simulink model "main"  (R2025b)
settings: Solver=ode4  StartTime=0.0  StopTime=60  FixedStep=Ts_inner  RelTol=1e-3
undefined symbols (not defined in the file): Ts_gcs
libraries: aerolibutil x4, instrumentseriallib x2, sldrtlib x1
settings Model: DataDictionary=project.sldd  Creator=Nick  LastModifiedBy=Nick
settings SolverCC: AutoInsertRateTranBlk=on

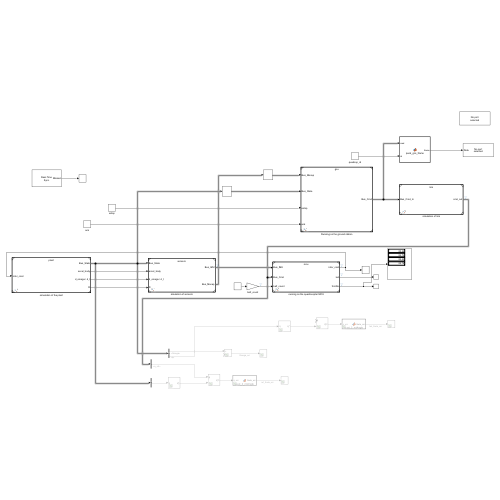
[thumbnail: Simulink's stored preview of the top-level diagram]
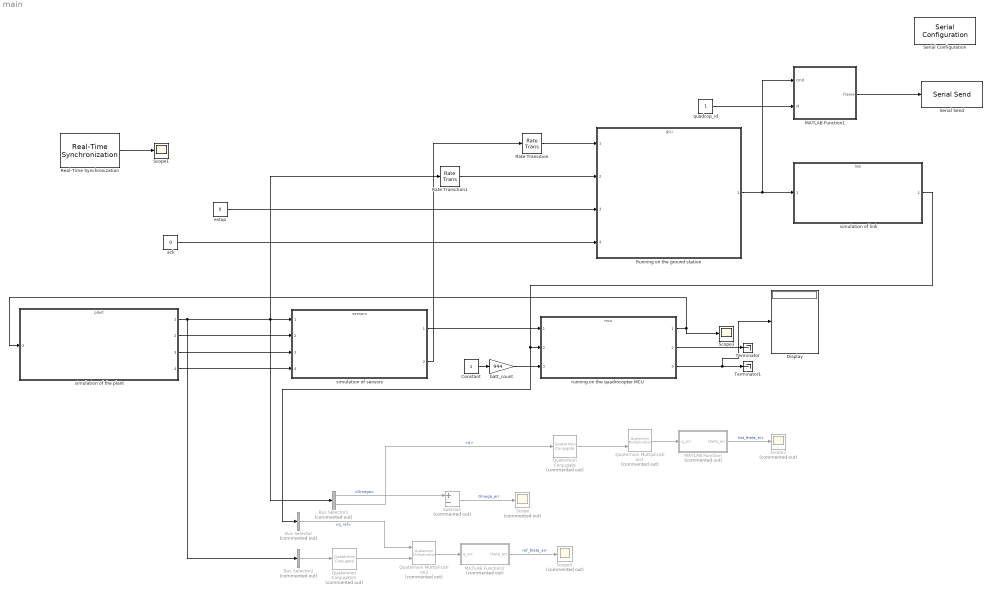
== system main ==
  Bus Selector : BusSelector  Commented=on  OutputSignals=q_ref
  Bus Selector1 : BusSelector  Commented=on  OutputSignals=Omega,q
  Bus Selector2 : BusSelector  Commented=on  OutputSignals=q  OutputAsBus=on
  Constant : Constant
  Display : Display
  MATLAB Function : MATLAB Function  Commented=on  TreatAsAtomicUnit=on
  MATLAB Function1 : MATLAB Function  TreatAsAtomicUnit=on
  MATLAB Function2 : MATLAB Function  Commented=on  TreatAsAtomicUnit=on
  Quaternion Conjugate : aerolibutil/Quaternion Conjugate  Commented=on
  Quaternion Conjugate1 : aerolibutil/Quaternion Conjugate  Commented=on
  Quaternion Multiplication1 : aerolibutil/Quaternion Multiplication  Commented=on
  Quaternion Multiplication2 : aerolibutil/Quaternion Multiplication  Commented=on
  Rate Transition : RateTransition  OutPortSampleTime=Ts_gcs
  Rate Transition1 : RateTransition  OutPortSampleTime=Ts_gcs
  Real-Time Synchronization : sldrtlib/Real-Time Synchronization  SampleTime=Ts_gcs  MaxMissedTicks=inf  ShowMissedTicks=on  YieldWhenWaiting=off
  Running on the ground station : ModelReference  ModelNameDialog=gcu.slx  SimulationMode=Normal  ModelReferenceVersion=1.298
  Scope : Scope  Commented=on
      settings: ActiveDisplayYMinimum=-1  ActiveDisplayYMaximum=1
  Scope1 : Scope
      settings: ActiveDisplayYMinimum=-1  ActiveDisplayYMaximum=1
  Scope2 : Scope  Commented=on
      settings: ActiveDisplayYMinimum=-0.084122920988905683  ActiveDisplayYMaximum=0.78039338720264007  DataLoggingVariableName=ScopeData2
  Scope3 : Scope
      settings: ActiveDisplayYMinimum=-656.76304621968529  ActiveDisplayYMaximum=5910.867415977169  DataLoggingVariableName=ScopeData3
  Scope5 : Scope  Commented=on
      settings: ActiveDisplayYMinimum=-0.013956380673274989  ActiveDisplayYMaximum=0.12560742605947492  DataLoggingVariableName=ScopeData5
  Serial Configuration : instrumentseriallib/Serial Configuration  Priority=-200000  PortSel=<Select a port...>  Port=<Select a port...>  ComPort=<Select a port...>  BaudRate=115200  DataBits=8  Parity=none  StopBits=1  ByteOrder=little-endian  FlowControl=none  Timeout=10  SimulateUsing=Interpreted execution  BlockInModel=on  aMode=1
      settings: LibrarySourceBlock=c2000lib/Host Communication/Serial Configuration
  Serial Send : instrumentseriallib/Serial Send  Priority=1  PortSel=<Select a port...>  Port=<Select a port...>  ComPort=<Select a port...>  Header=[]  Terminator=<none>  CustomTerminator=[]  EnableBlockingMode=on  SimulateUsing=Interpreted execution  BlockInModel=on  aMode=1
      settings: LibrarySourceBlock=c2000lib/Host Communication/Serial Send
  Subtract : Sum  Commented=on  Inputs=+-
  Terminator : Terminator
  Terminator1 : Terminator
  ack : Constant  Value=0  OutDataTypeStr=boolean
  batt_count : Gain  Gain=944
  estop : Constant  Value=0  OutDataTypeStr=uint8
  quadcop_id : Constant  OutDataTypeStr=uint8
  running on the quadrocopter MCU : ModelReference  ModelNameDialog=mcu.slx  SimulationMode=Normal  ModelReferenceVersion=1.269
  simulation of link : ModelReference  ModelNameDialog=link.slx  SimulationMode=Normal  ModelReferenceVersion=1.133
  simulation of sensors : ModelReference  ModelNameDialog=sensors.slx  SimulationMode=Normal  ModelReferenceVersion=1.85
  simulation of the plant : ModelReference  ModelNameDialog=plant.slx  SimulationMode=Normal  ModelReferenceVersion=1.208
  wires:
  simulation of the plant/1 -> Bus Selector2/1, Rate Transition1/1, Bus Selector1/1, simulation of sensors/1
  simulation of the plant/2 -> simulation of sensors/2
  simulation of the plant/3 -> simulation of sensors/3
  simulation of the plant/4 -> simulation of sensors/4
  simulation of sensors/1 -> running on the quadrocopter MCU/1
  simulation of sensors/2 -> Rate Transition/1
  Quaternion Conjugate/1 -> Quaternion Multiplication1/2
  MATLAB Function/1(theta_err) -> Scope2/1  "hat_theta_err"
  Quaternion Multiplication1/1 -> MATLAB Function/1(q_err)
  Bus Selector1/1 -> Subtract/1  "<Omega>"
  Subtract/1 -> Scope/1  "Omega_err"
  Bus Selector1/2 -> Quaternion Conjugate/1  "<q>"
  Bus Selector2/1 -> Quaternion Conjugate1/1
  Quaternion Multiplication2/1 -> MATLAB Function2/1(q_err)
  MATLAB Function2/1(theta_err) -> Scope5/1  "ref_theta_err"
  Quaternion Conjugate1/1 -> Quaternion Multiplication2/2
  Running on the ground station/1 -> MATLAB Function1/1(cmd), simulation of link/1
  Rate Transition/1 -> Running on the ground station/1
  Rate Transition1/1 -> Running on the ground station/2
  Bus Selector/1 -> Quaternion Multiplication2/1  "<q_ref>"
  simulation of link/1 -> Bus Selector/1, running on the quadrocopter MCU/2
  Real-Time Synchronization/1 -> Scope1/1
  estop/1 -> Running on the ground station/3
  ack/1 -> Running on the ground station/4
  Constant/1 -> batt_count/1
  batt_count/1 -> running on the quadrocopter MCU/3
  running on the quadrocopter MCU/1 -> Scope3/1, simulation of the plant/1
  running on the quadrocopter MCU/2 -> Terminator/1
  running on the quadrocopter MCU/3 -> Display/1, Terminator1/1
  quadcop_id/1 -> MATLAB Function1/2(id)
  MATLAB Function1/1(frame) -> Serial Send/1

== matlab function main/MATLAB Function ==
  data: q_err input; theta_err output
function theta_err = quat_2_rotAngle(q_err)   
%#codegen
    theta_err = 2*atan2(norm(q_err(2:4)), abs(q_err(1)));
end

== matlab function main/MATLAB Function2 ==
  data: q_err input; theta_err output
function theta_err = quat_2_rotAngle(q_err)   %#codegen
    theta_err = 2*atan2(norm(q_err(2:4)), abs(q_err(1)));
end

== matlab function main/MATLAB Function1 ==
  data: cmd input Bus: Bus_Cmd; frame output uint8 size=[1 82]; id input uint8 size=[1 1]
function frame = pack_gcs_frame(cmd, id)
%pack_gcs_frame  GS-USB-Frame [sync|id|Bus_Cmd(float32)|estop|ack|crc8] (82 B).
%   SSOT-Spiegel von gcs_frame.hpp (build). Zugleich die Byte-Spec fuer die
%   Simulink-Serial-Send-Seite
%
%   cmd: struct mit F_des, q_des(4), q_ref(4), Omega_ref(3), tau_ref(3),
%        q_ext(4), estop(0/1/2), ack(0/1). id: Ziel-Drohne (uint8, 0..15).
%   frame: 1x82 uint8, little-endian
%#codegen
    vals = single([ double(cmd.F_des); ...
                    reshape(double(cmd.q_des),4,1); ...
                    reshape(double(cmd.q_ref),4,1); ...
                    reshape(double(cmd.Omega_ref),3,1); ...
                    reshape(double(cmd.tau_ref),3,1); ...
                    reshape(double(cmd.q_ext),4,1) ]).'; % 1x19 single

    frame = zeros(1,82,'uint8');
    frame(1) = uint8(170); % 0xAA
    frame(2) = uint8(85); % 0x55
    frame(3) = uint8(id);
    frame(4:79) = typecast(vals, 'uint8'); % 19 x float32 = 76 Bytes
    frame(80) = uint8(cmd.estop);
    frame(81) = uint8(cmd.ack ~= 0);
    frame(82) = crc8(frame(3:81)); % über id + Payload + estop + ack
end

function c = crc8(bytes)
% CRC-8/SMBus: Poly 0x07, Init 0x00 (bitgleich zu gcs::detail::crc8).
    c = uint8(0);
    for k = 1:numel(bytes)
        c = bitxor(c, uint8(bytes(k)));
        for b = 1:8
            if bitand(c, uint8(128))
                c = bitxor(uint8(bitshift(c,1)), uint8(7));
            else
                c = uint8(bitshift(c,1));
            end
        end
    end
end
